simulink model "lista1_questao7"  (R2014b)
settings: Solver=ode45  StartTime=0.0  StopTime=92  RelTol=1e-3
libraries: cstblocks x5
settings Model: Creator=Danilo  LastModifiedBy=Danilo

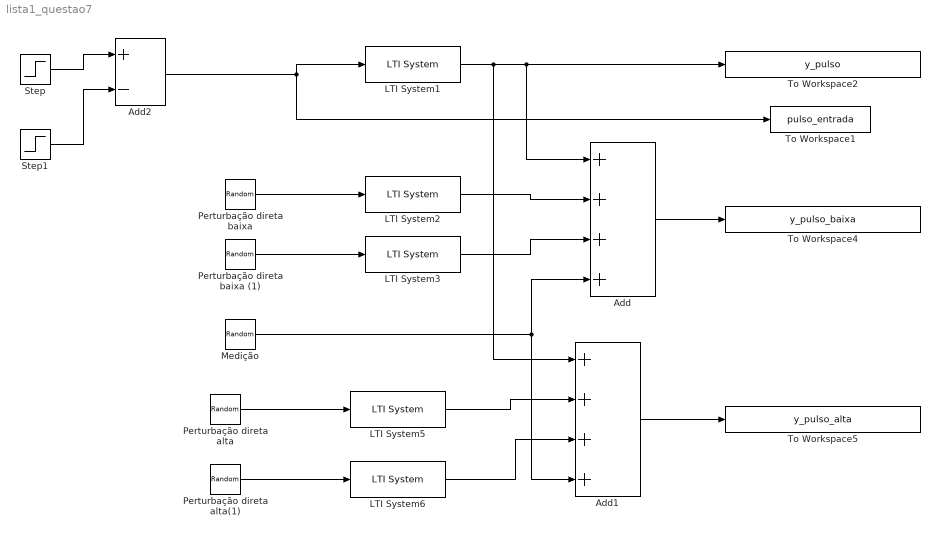
== system lista1_questao7 ==
  Add : Sum  Inputs=++++
  Add1 : Sum  Inputs=++++
  Add2 : Sum  Inputs=+-
  LTI System1 : cstblocks/LTI System  sys=H  IC=[]
  LTI System2 : cstblocks/LTI System  sys=G_pert_1  IC=[]
  LTI System3 : cstblocks/LTI System  sys=G_pert_2  IC=[]
  LTI System5 : cstblocks/LTI System  sys=G_pert_1  IC=[]
  LTI System6 : cstblocks/LTI System  sys=G_pert_2  IC=[]
  Medição : RandomNumber  Variance=exp(-6)  Seed=24  SampleTime=0.1
  Perturbação direta alta : RandomNumber  Variance=0.1  Seed=99  SampleTime=0.1
  Perturbação direta alta(1) : RandomNumber  Variance=0.1  Seed=22  SampleTime=0.1
  Perturbação direta baixa : RandomNumber  Variance=0.001  SampleTime=0.1
  Perturbação direta baixa (1) : RandomNumber  Variance=0.001  Seed=12  SampleTime=0.1
  Step : Step  Before=1  SampleTime=1
  Step1 : Step  SampleTime=1
  To Workspace1 : ToWorkspace  VariableName=pulso_entrada  SampleTime=1
  To Workspace2 : ToWorkspace  VariableName=y_pulso  SampleTime=1
  To Workspace4 : ToWorkspace  VariableName=y_pulso_baixa  SampleTime=1
  To Workspace5 : ToWorkspace  VariableName=y_pulso_alta  SampleTime=1
  wires:
  LTI System1/1 -> Add1/1, Add/1, To Workspace2/1
  Add/1 -> To Workspace4/1
  Perturbação direta baixa/1 -> LTI System2/1
  Perturbação direta baixa (1)/1 -> LTI System3/1
  LTI System2/1 -> Add/2
  LTI System3/1 -> Add/3
  Add1/1 -> To Workspace5/1
  Medição/1 -> Add/4, Add1/4
  Perturbação direta alta/1 -> LTI System5/1
  Perturbação direta alta(1)/1 -> LTI System6/1
  LTI System5/1 -> Add1/2
  LTI System6/1 -> Add1/3
  Add2/1 -> To Workspace1/1, LTI System1/1
  Step1/1 -> Add2/2
  Step/1 -> Add2/1
